simulink model "FOC_PI"  (R2024b)
settings: Solver=ode23tb  StartTime=0.0  StopTime=0.6  MaxStep=AUTO  RelTol=1e-4
InitFcn:
  | Ts=10e-6;
  | 
  | R=0.958;
  | Ld=5.25e-3;
  | Lq=12e-3;
  | Pn=4;
  | flux=0.1827;
libraries: slpidlib x3, spsPermanentMagnetSynchronousMachineLib x1, simulink x1, spsSVPWMGenerator2LevelLib x1, spsUniversalBridgeLib x1, spsDCVoltageSourceLib x1, sps_lib x1
settings Model: Creator=13524  LastModifiedBy=23954
settings SolverCC: ZeroCrossControl=DisableAll
settings RTWCC: GPUComputeCapability=3.5

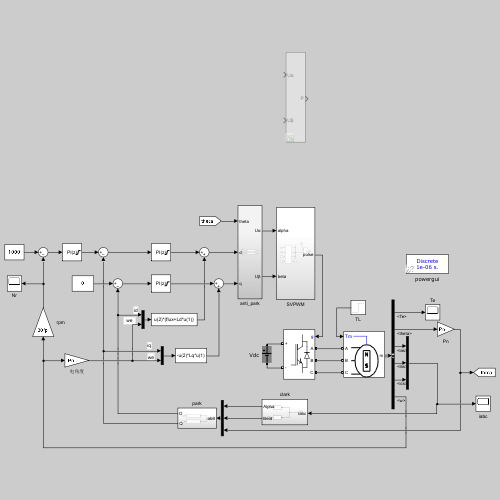
[thumbnail: Simulink's stored preview of the top-level diagram]
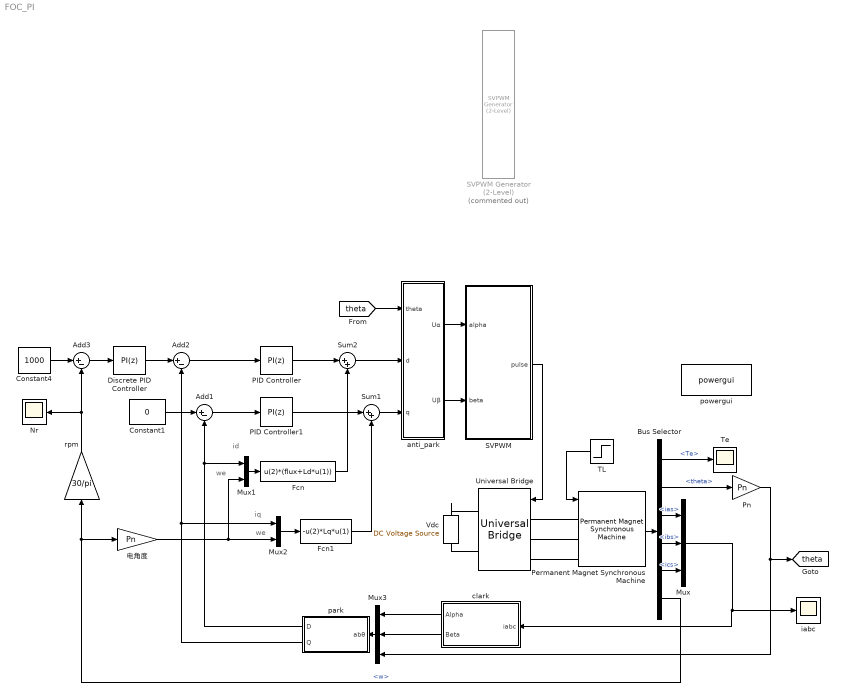
== system FOC_PI ==
  note: iq
  note: we
  note: we
  note: id
  Add1 : Sum  Inputs=|+-
  Add2 : Sum  Inputs=|+-
  Add3 : Sum  Inputs=|+-
  Bus Selector : BusSelector  OutputSignals=Te,theta,ias,ibs,ics,w
  Constant1 : Constant  Value=0
  Constant4 : Constant  Value=1000
  Discrete PID Controller : slpidlib/PID Controller  Controller=PI  Form=Ideal  TimeDomain=Discrete-time  UseExternalTs=off  SampleTime=Ts  IntegratorMethod=Forward Euler  FilterMethod=Forward Euler  ControllerParametersSource=internal  P=0.14  I=0.14*50  UseKiTs=off  D=0  UseExternalDerivativeSource=off  N=100  UseFilter=on  TunerSelectOption=Transfer Function Based (PID Tuner App)  InitialConditionSource=internal  InitialConditionForIntegrator=0  InitialConditionForFilter=0  DifferentiatorICPrevScaledInput=0  ExternalReset=none  TrackingMode=off  Kt=1  LimitOutput=on  SatLimitsSource=internal  UpperSaturationLimit=30  LowerSaturationLimit=-30  LinearizeAsGain=off  AntiWindupMode=none  Kb=1  LimitIntegrator=off  UpperIntegratorSaturationLimit=inf  LowerIntegratorSaturationLimit=-inf  POutMin=[]  POutMax=[]  IOutMin=[]  IOutMax=[]  DOutMin=[]  DOutMax=[]  NOutMin=[]  NOutMax=[]  SumOutMin=[]  SumOutMax=[]  SaturationOutMin=[]  SaturationOutMax=[]  PParamMin=[]  PParamMax=[]  IParamMin=[]  IParamMax=[]  DParamMin=[]  DParamMax=[]  NParamMin=[]  NParamMax=[]  KbParamMin=[]  KbParamMax=[]  KtParamMin=[]  KtParamMax=[]  KbOutMin=[]  KbOutMax=[]  KtOutMin=[]  KtOutMax=[]  IntegratorOutMin=[]  IntegratorOutMax=[]  FilterOutMin=[]  FilterOutMax=[]  SumI1OutMin=[]  SumI1OutMax=[]  SumI2OutMin=[]  SumI2OutMax=[]  SumI3OutMin=[]  SumI3OutMax=[]  SumI4OutMin=[]  SumI4OutMax=[]  SumDOutMin=[]  SumDOutMax=[]  DifferentiatorOutMin=[]  DifferentiatorOutMax=[]  FilterDiffOutCoefMin=[]  FilterDiffOutCoefMax=[]  ReciprocalOutMin=[]  ReciprocalOutMax=[]  SumDenOutMin=[]  SumDenOutMax=[]  SumNumOutMin=[]  SumNumOutMax=[]  DivideOutMin=[]  DivideOutMax=[]  UdiffTsProdOutMin=[]  UdiffTsProdOutMax=[]  NTsProdOutMin=[]  NTsProdOutMax=[]  UintegralTsProdOutMin=[]  UintegralTsProdOutMax=[]  UngainTsProdOutMin=[]  UngainTsProdOutMax=[]  ClampingZeroOutDataTypeStr=Inherit: Inherit via back propagation  ClampingZeroOutMin=[]  ClampingZeroOutMax=[]  FilterDenConstantOutDataTypeStr=Inherit: Inherit via back propagation  FilterDenConstantOutMin=[]  FilterDenConstantOutMax=[]  PCopyOutDataTypeStr=Inherit: Inherit via back propagation  PCopyOutMin=[]  PCopyOutMax=[]  NCopyOutDataTypeStr=Inherit: Inherit via back propagation  NCopyOutMin=[]  NCopyOutMax=[]  IntegratorContinuousStateAttributes=''  IntegratorStateMustResolveToSignalObject=off  IntegratorRTWStateStorageClass=Auto  FilterContinuousStateAttributes=''  FilterStateMustResolveToSignalObject=off  FilterRTWStateStorageClass=Auto  ParallelPVariant=Passthrough  IdealPVariant=InternalParameters  IVariant=InternalParameters  DVariant=Disabled  IntegratorVariant=Discrete  SatVariant=Enabled  AWVariant=Passthrough  PCopyVariant=Disabled  TRVariant=Disabled  FdbkBlocksVariant=Forward  IdealPFdbkVariant=Disabled  SatFdbkVariant=Disabled  DerivativeFilterVariant=Disabled  NVariant=Disabled  NCopyVariant=Disabled_SignalSpec  FilterICVariant=Disabled  IntegratorICVariant=InternalICs  ExternalResetVariant=Disabled  TRSumVariant=Passthrough  SumFdbkVariant=Disabled  SumVariant=Sum_PI  TsampFilterVariant=InternalTs  TsampNgainVariant=Passthrough  TsampIntegralVariant=Disabled_SignalSpec  ExternalSaturationOutDataTypeStr=Inherit: Same as second input  DerivativeSourceVariant=Disabled  PreIntVariant=InternalPreInt
      settings: LibrarySourceBlock=simulink/Discrete/Discrete PID Controller
  Fcn : Fcn  Expr=u(2)*(flux+Ld*u(1))
  Fcn1 : Fcn  Expr=-u(2)*Lq*u(1)
  Mux : Mux  Inputs=3
  Mux1 : Mux  Inputs=2
  Mux2 : Mux  Inputs=2
  Mux3 : Mux  Inputs=3
  Nr : Scope
  PID Controller : slpidlib/PID Controller  Controller=PI  Form=Parallel  TimeDomain=Discrete-time  UseExternalTs=off  SampleTime=Ts  IntegratorMethod=Forward Euler  FilterMethod=Forward Euler  ControllerParametersSource=internal  P=Lq*1100  I=R*1100  UseKiTs=off  D=0  UseExternalDerivativeSource=off  N=100  UseFilter=on  TunerSelectOption=Transfer Function Based (PID Tuner App)  InitialConditionSource=internal  InitialConditionForIntegrator=0  InitialConditionForFilter=0  DifferentiatorICPrevScaledInput=0  ExternalReset=none  TrackingMode=off  Kt=1  LimitOutput=on  SatLimitsSource=internal  UpperSaturationLimit=311*0.9*sqrt(1/3)  LowerSaturationLimit=-311*0.9*sqrt(1/3)  LinearizeAsGain=on  AntiWindupMode=none  Kb=1  LimitIntegrator=off  UpperIntegratorSaturationLimit=inf  LowerIntegratorSaturationLimit=-inf  POutMin=[]  POutMax=[]  IOutMin=[]  IOutMax=[]  DOutMin=[]  DOutMax=[]  NOutMin=[]  NOutMax=[]  SumOutMin=[]  SumOutMax=[]  SaturationOutMin=[]  SaturationOutMax=[]  PParamMin=[]  PParamMax=[]  IParamMin=[]  IParamMax=[]  DParamMin=[]  DParamMax=[]  NParamMin=[]  NParamMax=[]  KbParamMin=[]  KbParamMax=[]  KtParamMin=[]  KtParamMax=[]  KbOutMin=[]  KbOutMax=[]  KtOutMin=[]  KtOutMax=[]  IntegratorOutMin=[]  IntegratorOutMax=[]  FilterOutMin=[]  FilterOutMax=[]  SumI1OutMin=[]  SumI1OutMax=[]  SumI2OutMin=[]  SumI2OutMax=[]  SumI3OutMin=[]  SumI3OutMax=[]  SumI4OutMin=[]  SumI4OutMax=[]  SumDOutMin=[]  SumDOutMax=[]  DifferentiatorOutMin=[]  DifferentiatorOutMax=[]  FilterDiffOutCoefMin=[]  FilterDiffOutCoefMax=[]  ReciprocalOutMin=[]  ReciprocalOutMax=[]  SumDenOutMin=[]  SumDenOutMax=[]  SumNumOutMin=[]  SumNumOutMax=[]  DivideOutMin=[]  DivideOutMax=[]  UdiffTsProdOutMin=[]  UdiffTsProdOutMax=[]  NTsProdOutMin=[]  NTsProdOutMax=[]  UintegralTsProdOutMin=[]  UintegralTsProdOutMax=[]  UngainTsProdOutMin=[]  UngainTsProdOutMax=[]  ClampingZeroOutDataTypeStr=Inherit: Inherit via back propagation  ClampingZeroOutMin=[]  ClampingZeroOutMax=[]  FilterDenConstantOutDataTypeStr=Inherit: Inherit via back propagation  FilterDenConstantOutMin=[]  FilterDenConstantOutMax=[]  PCopyOutDataTypeStr=Inherit: Inherit via back propagation  PCopyOutMin=[]  PCopyOutMax=[]  NCopyOutDataTypeStr=Inherit: Inherit via back propagation  NCopyOutMin=[]  NCopyOutMax=[]  IntegratorContinuousStateAttributes=''  IntegratorStateMustResolveToSignalObject=off  IntegratorRTWStateStorageClass=Auto  FilterContinuousStateAttributes=''  FilterStateMustResolveToSignalObject=off  FilterRTWStateStorageClass=Auto  ParallelPVariant=InternalParameters  IdealPVariant=Disabled  IVariant=InternalParameters  DVariant=Disabled  IntegratorVariant=Discrete  SatVariant=Enabled  AWVariant=Passthrough  PCopyVariant=Disabled  TRVariant=Disabled  FdbkBlocksVariant=Forward  IdealPFdbkVariant=Disabled  SatFdbkVariant=Disabled  DerivativeFilterVariant=Disabled  NVariant=Disabled  NCopyVariant=Disabled_SignalSpec  FilterICVariant=Disabled  IntegratorICVariant=InternalICs  ExternalResetVariant=Disabled  TRSumVariant=Passthrough  SumFdbkVariant=Disabled  SumVariant=Sum_PI  TsampFilterVariant=InternalTs  TsampNgainVariant=Passthrough  TsampIntegralVariant=Disabled_SignalSpec  ExternalSaturationOutDataTypeStr=Inherit: Same as second input  DerivativeSourceVariant=Disabled  PreIntVariant=InternalPreInt
  PID Controller1 : slpidlib/PID Controller  Controller=PI  Form=Parallel  TimeDomain=Discrete-time  UseExternalTs=off  SampleTime=Ts  IntegratorMethod=Forward Euler  FilterMethod=Forward Euler  ControllerParametersSource=internal  P=Ld*1100  I=R*1100  UseKiTs=off  D=0  UseExternalDerivativeSource=off  N=100  UseFilter=on  TunerSelectOption=Transfer Function Based (PID Tuner App)  InitialConditionSource=internal  InitialConditionForIntegrator=0  InitialConditionForFilter=0  DifferentiatorICPrevScaledInput=0  ExternalReset=none  TrackingMode=off  Kt=1  LimitOutput=on  SatLimitsSource=internal  UpperSaturationLimit=311*0.9*sqrt(1/3)  LowerSaturationLimit=-311*0.9*sqrt(1/3)  LinearizeAsGain=on  AntiWindupMode=none  Kb=1  LimitIntegrator=off  UpperIntegratorSaturationLimit=inf  LowerIntegratorSaturationLimit=-inf  POutMin=[]  POutMax=[]  IOutMin=[]  IOutMax=[]  DOutMin=[]  DOutMax=[]  NOutMin=[]  NOutMax=[]  SumOutMin=[]  SumOutMax=[]  SaturationOutMin=[]  SaturationOutMax=[]  PParamMin=[]  PParamMax=[]  IParamMin=[]  IParamMax=[]  DParamMin=[]  DParamMax=[]  NParamMin=[]  NParamMax=[]  KbParamMin=[]  KbParamMax=[]  KtParamMin=[]  KtParamMax=[]  KbOutMin=[]  KbOutMax=[]  KtOutMin=[]  KtOutMax=[]  IntegratorOutMin=[]  IntegratorOutMax=[]  FilterOutMin=[]  FilterOutMax=[]  SumI1OutMin=[]  SumI1OutMax=[]  SumI2OutMin=[]  SumI2OutMax=[]  SumI3OutMin=[]  SumI3OutMax=[]  SumI4OutMin=[]  SumI4OutMax=[]  SumDOutMin=[]  SumDOutMax=[]  DifferentiatorOutMin=[]  DifferentiatorOutMax=[]  FilterDiffOutCoefMin=[]  FilterDiffOutCoefMax=[]  ReciprocalOutMin=[]  ReciprocalOutMax=[]  SumDenOutMin=[]  SumDenOutMax=[]  SumNumOutMin=[]  SumNumOutMax=[]  DivideOutMin=[]  DivideOutMax=[]  UdiffTsProdOutMin=[]  UdiffTsProdOutMax=[]  NTsProdOutMin=[]  NTsProdOutMax=[]  UintegralTsProdOutMin=[]  UintegralTsProdOutMax=[]  UngainTsProdOutMin=[]  UngainTsProdOutMax=[]  ClampingZeroOutDataTypeStr=Inherit: Inherit via back propagation  ClampingZeroOutMin=[]  ClampingZeroOutMax=[]  FilterDenConstantOutDataTypeStr=Inherit: Inherit via back propagation  FilterDenConstantOutMin=[]  FilterDenConstantOutMax=[]  PCopyOutDataTypeStr=Inherit: Inherit via back propagation  PCopyOutMin=[]  PCopyOutMax=[]  NCopyOutDataTypeStr=Inherit: Inherit via back propagation  NCopyOutMin=[]  NCopyOutMax=[]  IntegratorContinuousStateAttributes=''  IntegratorStateMustResolveToSignalObject=off  IntegratorRTWStateStorageClass=Auto  FilterContinuousStateAttributes=''  FilterStateMustResolveToSignalObject=off  FilterRTWStateStorageClass=Auto  ParallelPVariant=InternalParameters  IdealPVariant=Disabled  IVariant=InternalParameters  DVariant=Disabled  IntegratorVariant=Discrete  SatVariant=Enabled  AWVariant=Passthrough  PCopyVariant=Disabled  TRVariant=Disabled  FdbkBlocksVariant=Forward  IdealPFdbkVariant=Disabled  SatFdbkVariant=Disabled  DerivativeFilterVariant=Disabled  NVariant=Disabled  NCopyVariant=Disabled_SignalSpec  FilterICVariant=Disabled  IntegratorICVariant=InternalICs  ExternalResetVariant=Disabled  TRSumVariant=Passthrough  SumFdbkVariant=Disabled  SumVariant=Sum_PI  TsampFilterVariant=InternalTs  TsampNgainVariant=Passthrough  TsampIntegralVariant=Disabled_SignalSpec  ExternalSaturationOutDataTypeStr=Inherit: Same as second input  DerivativeSourceVariant=Disabled  PreIntVariant=InternalPreInt
  Permanent Magnet Synchronous Machine : spsPermanentMagnetSynchronousMachineLib/Permanent Magnet Synchronous Machine  NbPhases=3  FluxDistribution=Sinusoidal  RotorType=Salient-pole  MechanicalLoad=Torque Tm  PresetModel=No  ShowDetailedParameters=on  MeasurementBus=on  Resistance=0.958  Inductance=8.5e-3  dqInductances=[5.25e-3,12e-3]  La=0.00525  MachineConstant=Flux linkage established by magnets (V.s)  Flux=0.1827  VoltageCst=132.5525  TorqueCst=1.0962  Flat=120  Mechanical=[0.003 0.008 4 0]  PolePairs=4  InitialConditions=[0,0, 0,0]  InitialConditions5ph=[0 0 0 0 0 0]  RefAngle=Aligned with phase A axis (original Park)  IterativeDiscreteModel=Trapezoidal non iterative  TsBlock=-1  TsPowergui=0
  Pn : Gain  Gain=Pn
  SVPWM : Subsystem
  SVPWM Generator (2-Level) : spsSVPWMGenerator2LevelLib/SVPWM Generator (2-Level)  Commented=on  InputType=alpha-beta components  SwitchingPattern=Pattern #1  Fc=1/0.0001  ParUref=[0.8 -30 50]  Ts=0
  Sum1 : Sum  Inputs=|++
  Sum2 : Sum  Inputs=|++
  TL : Step  Time=0.2  After=10  SampleTime=0
  Te : Scope
  Universal Bridge : spsUniversalBridgeLib/Universal Bridge  Arms=3  SnubberResistance=1e5  SnubberCapacitance=inf  Device=IGBT / Diodes  Ron=1e-3  Lon=0  ForwardVoltages="[  0  0  ]"  ForwardVoltage=0  GTOparameters=[ 10e-6 , 20e-6 ]  IGBTparameters=[ 1e-6 , 2e-6 ]  Measurements=None  Measurements_2=None  converterType=Rectifier
  Vdc : spsDCVoltageSourceLib/DC Voltage Source  Amplitude=311  Measurements=None
  anti_park : Subsystem
  clark : Subsystem
  iabc : Scope
  park : Subsystem
  powergui : sps_lib/powergui  SimulationMode=Discrete  SampleTime=10e-7  frequency=60  Iterations=50  frequencyindice=0  Pbase=100e6  ErrMax=1e-4  UnitsV=kV  UnitsW=MW  buscounter=0  FunctionMessages=off  echomessages=off  EnableUseOfTLC=off  CurrentSourceSwitches=off  DisableSnubberDevices=off  DisableRonSwitches=off  DisableVfSwitches=off  DisplayEquations=off  AutomaticDiscreteSolvers=off  SolverType=Tustin/Backward Euler (TBE)  Interpol=off  ExternalGateDelay=off  methode=off  Ts=0  x0status=blocks  SPID=off  SwTol=0  HookPort=off  NonlinearTolerance=1e-4  nMaxIteration=100  ContinueOnMaxIteration=off  RestoreLinks=warning  ResistiveCurrentMeasurement=off  Frange=[0:2:500]  Ylog=off  Xlog=on  ShowGrid=off  save=off  variable=ZData  structure=0  ZoomFFT=on  StartTime=0.0  cycles=1  DisplayStyle=1  fundamental=60  FreqAxis=off  MaxFrequency=1000  frequencyindicesteady=1  RmsSteady=1  display=off
  rpm : Gain  Gain=30/pi
  电角度 : Gain  Gain=Pn
  tag scope: theta=global
  wires:
  Fcn1/1 -> Sum1/2
  PID Controller1/1 -> Sum1/1
  Pn/1 -> Mux3/3, [theta]
  Fcn/1 -> Sum2/2
  Constant1/1 -> Add1/1
  Add1/1 -> PID Controller1/1
  Mux2/1 -> Fcn1/1
  Bus Selector/1 -> Te/1  "<Te>"
  Bus Selector/6 -> 电角度/1, rpm/1  "<w>"
  rpm/1 -> Add3/2, Nr/1
  PID Controller/1 -> Sum2/1
  电角度/1 -> Mux2/2, Mux1/2
  Mux/1 -> clark/1(iabc), iabc/1
  Bus Selector/2 -> Pn/1  "<theta>"
  TL/1 -> Permanent Magnet Synchronous Machine/1
  Add3/1 -> Discrete PID Controller/1
  Constant4/1 -> Add3/1
  park/1(D) -> Mux1/1, Add1/2
  Mux1/1 -> Fcn/1
  Add2/1 -> PID Controller/1
  park/2(Q) -> Mux2/1, Add2/2
  Discrete PID Controller/1 -> Add2/1
  clark/1(Alpha) -> Mux3/1
  clark/2(Beta) -> Mux3/2
  Mux3/1 -> park/1(abθ)
  Sum1/1 -> anti_park/3(q)
  Sum2/1 -> anti_park/2(d)
  [theta] -> anti_park/1(theta)
  Permanent Magnet Synchronous Machine/1 -> Bus Selector/1
  Bus Selector/3 -> Mux/1  "<ias>"
  Bus Selector/4 -> Mux/2  "<ibs>"
  Bus Selector/5 -> Mux/3  "<ics>"
  anti_park/2(Uβ) -> SVPWM/2(beta)
  anti_park/1(Uα) -> SVPWM/1(alpha)
  SVPWM/1(pulse) -> Universal Bridge/1
  connections:
  Universal Bridge/LConn2 -- Permanent Magnet Synchronous Machine/LConn2
  Universal Bridge/LConn3 -- Permanent Magnet Synchronous Machine/LConn3
  Vdc/RConn1 -- Universal Bridge/RConn1
  Universal Bridge/RConn2 -- Vdc/LConn1
  Universal Bridge/LConn1 -- Permanent Magnet Synchronous Machine/LConn1

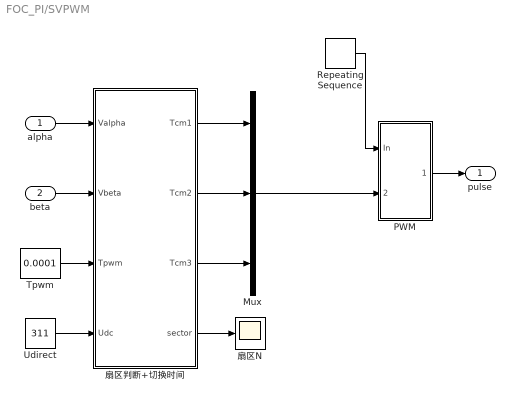
== system FOC_PI/SVPWM ==
  alpha : Inport
  beta : Inport  Port=2
  Mux : Mux  Inputs=3
  PWM : Subsystem
  Repeating Sequence : simulink/Sources/Repeating Sequence  rep_seq_t=[0 0.00005 0.0001]  rep_seq_y=[0 0.00005 0]
  Tpwm : Constant  Value=0.0001
  Udirect : Constant  Value=311
  扇区N : Scope
  扇区判断+切换时间 : MATLAB Function  TreatAsAtomicUnit=on
  pulse : Outport
  wires:
  alpha/1 -> 扇区判断+切换时间/1(Valpha)
  beta/1 -> 扇区判断+切换时间/2(Vbeta)
  Tpwm/1 -> 扇区判断+切换时间/3(Tpwm)
  Udirect/1 -> 扇区判断+切换时间/4(Udc)
  扇区判断+切换时间/4(sector) -> 扇区N/1
  Mux/1 -> PWM/2(Tcm123)
  PWM/1(PWM) -> pulse/1
  Repeating Sequence/1 -> PWM/1(In)
  扇区判断+切换时间/2(Tcm2) -> Mux/2
  扇区判断+切换时间/1(Tcm1) -> Mux/1
  扇区判断+切换时间/3(Tcm3) -> Mux/3

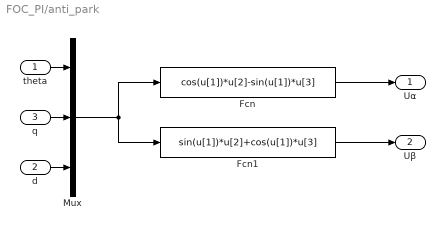
== system FOC_PI/anti_park ==
  theta : Inport
  d : Inport  Port=2
  q : Inport  Port=3
  Fcn : Fcn  Expr=cos(u[1])*u[2]-sin(u[1])*u[3]
  Fcn1 : Fcn  Expr=sin(u[1])*u[2]+cos(u[1])*u[3]
  Mux : Mux  Inputs=3
  Uα : Outport
  Uβ : Outport  Port=2
  wires:
  Fcn/1 -> Uα/1
  Fcn1/1 -> Uβ/1
  theta/1 -> Mux/1
  Mux/1 -> Fcn1/1, Fcn/1
  q/1 -> Mux/2
  d/1 -> Mux/3

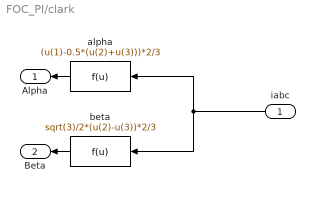
== system FOC_PI/clark ==
  iabc : Inport
  alpha : Fcn  Expr=(u(1)-0.5*(u(2)+u(3)))*2/3
  beta : Fcn  Expr=sqrt(3)/2*(u(2)-u(3))*2/3
  Alpha : Outport
  Beta : Outport  Port=2
  wires:
  iabc/1 -> alpha/1, beta/1
  alpha/1 -> Alpha/1
  beta/1 -> Beta/1

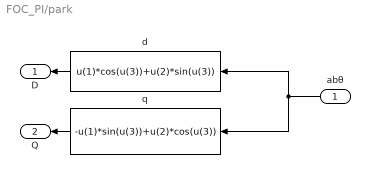
== system FOC_PI/park ==
  abθ : Inport
  d : Fcn  Expr=u(1)*cos(u(3))+u(2)*sin(u(3))
  q : Fcn  Expr=-u(1)*sin(u(3))+u(2)*cos(u(3))
  D : Outport
  Q : Outport  Port=2
  wires:
  q/1 -> Q/1
  d/1 -> D/1
  abθ/1 -> q/1, d/1

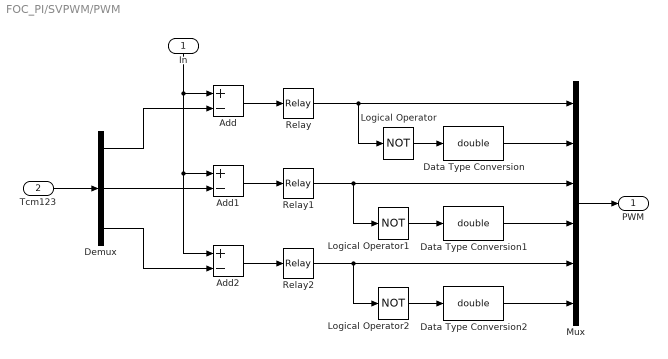
== system FOC_PI/SVPWM/PWM ==
  In : Inport
  Tcm123 : Inport  Port=2
  Add : Sum  Inputs=+-
  Add1 : Sum  Inputs=+-
  Add2 : Sum  Inputs=+-
  Data Type Conversion : DataTypeConversion  OutDataTypeStr=double  SaturateOnIntegerOverflow=off  RndMeth=Floor
  Data Type Conversion1 : DataTypeConversion  OutDataTypeStr=double  SaturateOnIntegerOverflow=off  RndMeth=Floor
  Data Type Conversion2 : DataTypeConversion  OutDataTypeStr=double  SaturateOnIntegerOverflow=off  RndMeth=Floor
  Demux : Demux  Outputs=3
  Logical Operator : Logic  Operator=NOT  AllPortsSameDT=off  OutDataTypeStr=boolean
  Logical Operator1 : Logic  Operator=NOT  AllPortsSameDT=off  OutDataTypeStr=boolean
  Logical Operator2 : Logic  Operator=NOT  AllPortsSameDT=off  OutDataTypeStr=boolean
  Mux : Mux  Inputs=6
  Relay : Relay  OffSwitchValue=-eps
  Relay1 : Relay  OffSwitchValue=-eps
  Relay2 : Relay  OffSwitchValue=-eps
  PWM : Outport
  wires:
  Demux/3 -> Add2/2
  Demux/2 -> Add1/2
  Demux/1 -> Add/2
  Relay2/1 -> Mux/5, Logical Operator2/1
  Relay1/1 -> Mux/3, Logical Operator1/1
  Relay/1 -> Logical Operator/1, Mux/1
  Mux/1 -> PWM/1
  Data Type Conversion/1 -> Mux/2
  Data Type Conversion1/1 -> Mux/4
  Data Type Conversion2/1 -> Mux/6
  Logical Operator2/1 -> Data Type Conversion2/1
  Logical Operator1/1 -> Data Type Conversion1/1
  Logical Operator/1 -> Data Type Conversion/1
  Add1/1 -> Relay1/1
  Add2/1 -> Relay2/1
  Add/1 -> Relay/1
  In/1 -> Add/1, Add2/1, Add1/1
  Tcm123/1 -> Demux/1

== matlab function FOC_PI/SVPWM/扇区判断+切换时间 ==
  data: Valpha input; Tcm1 output; Vbeta input; Tpwm input; Udc input; Tcm2 output; Tcm3 output; sector output
function [ Tcm1, Tcm2,  Tcm3,  sector] = fcn(Valpha, Vbeta, Tpwm, Udc)

% #codegen
%变量初始化
sector = 0;
Tcm1 = 0;
Tcm2 = 0;
Tcm3 = 0;
% = = = = = = = = Parameters statement = = = = = = = = = = = = = = = =
%P37 2-18

Vref1 = Vbeta;
Vref2 = ( sqrt(3)*Valpha- Vbeta) / 2;
Vref3 = ( -sqrt(3)*Valpha- Vbeta) / 2;
%＝= = = = = = = Sector calculation=================
%扇区判断
if  (Vref1> 0)
    sector = 1;
end
if  (Vref2> 0)
    sector = sector + 2;
end
if (Vref3> 0)
    sector = sector + 4;
end


%＝＝＝＝＝＝＝＝ X Y Z calculation===================
%P38 2-21

X = sqrt(3) * Vbeta * Tpwm/Udc;
Y = Tpwm/Udc * (3/2 *Valpha + sqrt(3)/2 * Vbeta);
Z = Tpwm/Udc * (-3/2 * Valpha + sqrt(3)/2 * Vbeta);

% = = = =======Duty ratio calculation================
%根据表2-5计算

switch (sector)
    case 1
        T1 = Z; T2 = Y;
    case 2
        T1 = Y; T2 = - X;
    case 3
        T1 = -Z; T2 = X;
    case 4
        T1 = -X; T2 = Z;
    case 5
        T1 = X; T2 = -Y;
    otherwise
        T1 = -Y; T2 = -Z;
end
%过调制处理
if T1 + T2 > Tpwm
    T1 = T1/(T1 + T2);
    T2 = T2/(T1+ T2);
else
    T1 = T1;
    T2 = T2;
end

ta= (Tpwm -(T1+T2))/ 4.0;
tb = ta+ T1/ 2;
tc = tb + T2/ 2;

%＝= = =======Duty ratio calculation================
%根据表2-6计算 各扇区时间切换点
switch (sector)
    case 1
        Tcm1 = tb;
        Tcm2 = ta;
        Tcm3 = tc;
    case 2
        Tcm1 = ta;
        Tcm2 = tc;
        Tcm3 = tb;
    case 3
        Tcm1 = ta;
        Tcm2 = tb;
        Tcm3 = tc;
    case 4
        Tcm1 = tc;
        Tcm2 = tb;
        Tcm3 = ta;
    case 5
        Tcm1 = tc;
        Tcm2 = ta;
        Tcm3 = tb;
    case 6
        Tcm1 = tb;
        Tcm2 = tc;
        Tcm3 = ta;
end
end
